simulink model "SERVER"  (R2021a)
settings: Solver=FixedStepDiscrete  StartTime=0.0  StopTime=inf  FixedStep=0.01  RelTol=1e-3  EnableMultiTasking=on
libraries: arduinolib x9, simulink x3, canmsglib x2, simulink_extras x1, dspswit3 x1
settings Model: SimulationMode=external  SILPILModeSetting=veronly  ExtModeEnableFloating=off  ExtModeTrigDuration=2  ExtModeTrigDurationFloating=2  Creator=Le Thanh Tu  LastModifiedBy=Le Thanh Tu
settings SolverCC: AlgebraicLoopSolver=TrustRegion  PositivePriorityOrder=on  AutoInsertRateTranBlk=on
settings DataIOCC: ExternalInput=[value]  SaveOutput=off  SignalLogging=off  DSMLogging=off  SaveTime=off  ReturnWorkspaceOutputs=off
settings OptimizationCC: EnhancedBackFolding=on  PassReuseOutputArgsAs=Individual arguments  ZeroExternalMemoryAtStartup=off  ZeroInternalMemoryAtStartup=off  MaxStackSize=64  OptimizeBlockOrder=speed  DifferentSizesBufferReuse=on  OptimizationCustomize=off  EfficientTunableParamExpr=on
settings DebuggingCC: ParameterTunabilityLossMsg=error  SFMachineParentedDataDiag=warning
settings HardwareCC: ProdBitPerPointer=32  ProdBitPerSizeT=32  ProdBitPerPtrDiffT=32  ProdLargestAtomicInteger=Long  ProdLargestAtomicFloat=Double  ProdWordSize=32  ProdHWDeviceType=ARM Compatible->ARM Cortex
settings SFSimCC: MATLABDynamicMemAlloc=off
settings RTWCC: SystemTargetFile=ert.tlc  HardwareBoard=Arduino Due  TemplateMakefile=ert_default_tmf  RetainRTWFile=on  Toolchain=Arduino ARM  BuildConfiguration=Faster Runs
settings CodeAppCC: ForceParamTrailComments=on  IgnoreCustomStorageClasses=off  OperatorAnnotations=on  SimulinkDataObjDesc=on  SFDataObjDesc=on  InsertBlockDesc=on
settings ERTTargetCC: SupportContinuousTime=on  SupportVariableSizeSignals=on  ExtModeStaticAllocSize=24576

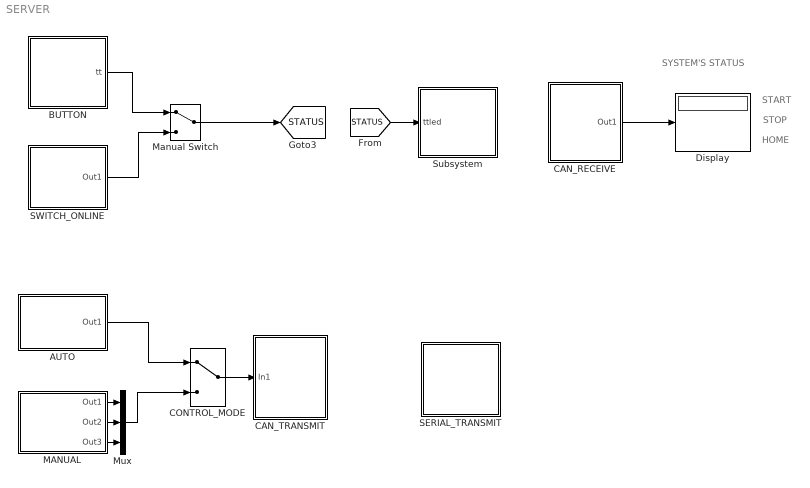
== system SERVER ==
  note: SYSTEM'S STATUS
  note: START
  note: STOP
  note: HOME
  AUTO : Subsystem
  BUTTON : Subsystem
  CAN_RECEIVE : Subsystem
  CAN_TRANSMIT : Subsystem
  CONTROL_MODE : ManualSwitch
  Display : Display
      settings: Decimation=3
  MANUAL : Subsystem
  Manual Switch : ManualSwitch
  Mux : Mux  Inputs=3
  SERIAL_TRANSMIT : Subsystem
  SWITCH_ONLINE : Subsystem
  Subsystem : Subsystem
  tag scope: STATUS=global
  wires:
  MANUAL/1(Out1) -> Mux/1
  MANUAL/2(Out2) -> Mux/2
  MANUAL/3(Out3) -> Mux/3
  Mux/1 -> CONTROL_MODE/2
  AUTO/1(Out1) -> CONTROL_MODE/1
  CAN_RECEIVE/1(Out1) -> Display/1
  SWITCH_ONLINE/1(Out1) -> Manual Switch/2
  Manual Switch/1 -> [STATUS]
  BUTTON/1(tt) -> Manual Switch/1
  CONTROL_MODE/1 -> CAN_TRANSMIT/1(In1)
  [STATUS] -> Subsystem/1(ttled)

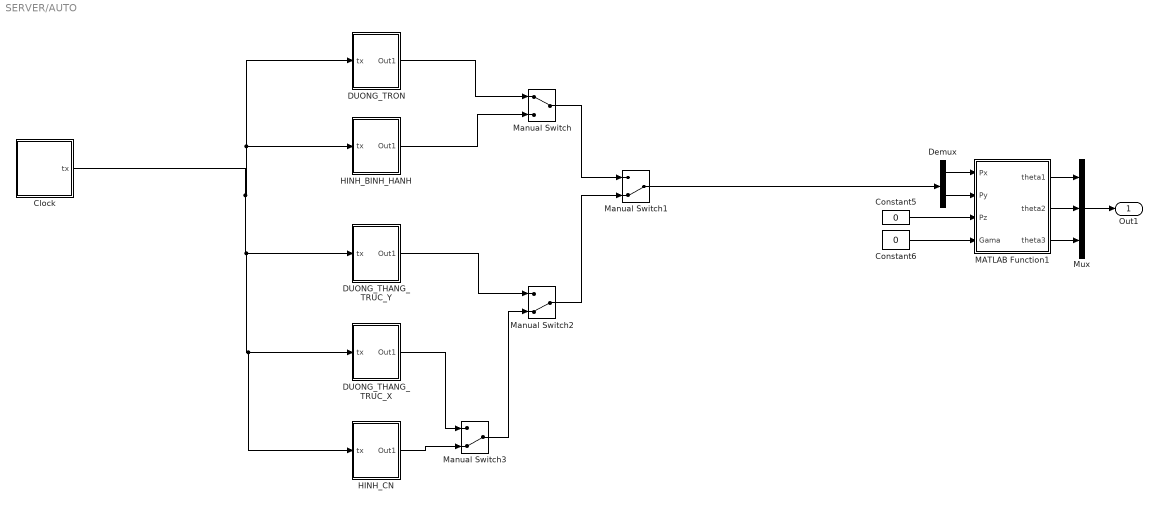
== system SERVER/AUTO ==
  Clock : Subsystem
  Constant5 : Constant  Value=0
  Constant6 : Constant  Value=0
  DUONG_THANG_TRUC_X : Subsystem
  DUONG_THANG_TRUC_Y : Subsystem
  DUONG_TRON : Subsystem
  Demux : Demux  Outputs=2
  HINH_BINH_HANH : Subsystem
  HINH_CN : Subsystem
  MATLAB Function1 : MATLAB Function  TreatAsAtomicUnit=on
  Manual Switch : ManualSwitch
  Manual Switch1 : ManualSwitch  CurrentSetting=0
  Manual Switch2 : ManualSwitch  CurrentSetting=0
  Manual Switch3 : ManualSwitch  CurrentSetting=0
  Mux : Mux  Inputs=3
  Out1 : Outport
  wires:
  HINH_BINH_HANH/1(Out1) -> Manual Switch/2
  Manual Switch2/1 -> Manual Switch1/2
  Manual Switch/1 -> Manual Switch1/1
  Demux/2 -> MATLAB Function1/2(Py)
  MATLAB Function1/3(theta3) -> Mux/3
  Demux/1 -> MATLAB Function1/1(Px)
  DUONG_TRON/1(Out1) -> Manual Switch/1
  Mux/1 -> Out1/1
  MATLAB Function1/1(theta1) -> Mux/1
  Constant5/1 -> MATLAB Function1/3(Pz)
  DUONG_THANG_TRUC_Y/1(Out1) -> Manual Switch2/1
  Constant6/1 -> MATLAB Function1/4(Gama)
  Manual Switch1/1 -> Demux/1
  MATLAB Function1/2(theta2) -> Mux/2
  Clock/1(tx) -> HINH_CN/1(tx), DUONG_THANG_TRUC_X/1(tx), DUONG_THANG_TRUC_Y/1(tx), HINH_BINH_HANH/1(tx), DUONG_TRON/1(tx)
  DUONG_THANG_TRUC_X/1(Out1) -> Manual Switch3/1
  Manual Switch3/1 -> Manual Switch2/2
  HINH_CN/1(Out1) -> Manual Switch3/2

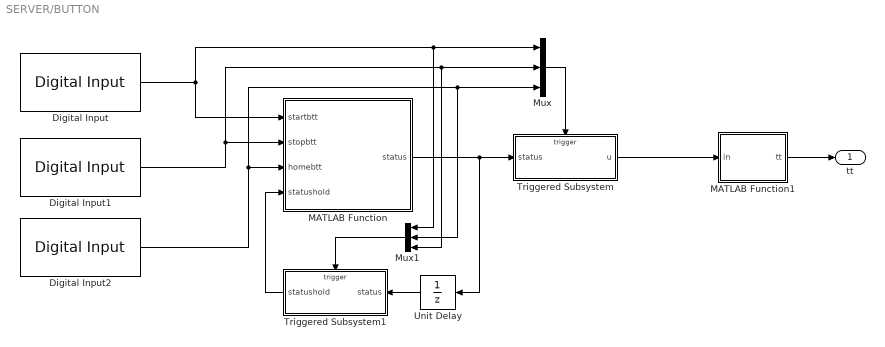
== system SERVER/BUTTON ==
  Digital Input : arduinolib/Digital Input  pinNumber=16  mode=Default  Direction=input  SampleTime=0.01  blockPlatform=arduino
  Digital Input1 : arduinolib/Digital Input  pinNumber=17  mode=Default  Direction=input  SampleTime=0.01  blockPlatform=arduino
  Digital Input2 : arduinolib/Digital Input  pinNumber=18  mode=Default  Direction=input  SampleTime=0.01  blockPlatform=arduino
  MATLAB Function : MATLAB Function  TreatAsAtomicUnit=on
  MATLAB Function1 : MATLAB Function  TreatAsAtomicUnit=on
  Mux : Mux  Inputs=3
  Mux1 : Mux  Inputs=3
  Triggered Subsystem : Subsystem  TreatAsAtomicUnit=on
  Triggered Subsystem1 : Subsystem  TreatAsAtomicUnit=on
  Unit Delay : UnitDelay  SampleTime=-1  HasFrameUpgradeWarning=on
  tt : Outport
  wires:
  Triggered Subsystem/1(u) -> MATLAB Function1/1(in)
  Digital Input2/1 -> MATLAB Function/3(homebtt), Mux1/2, Mux/3
  Unit Delay/1 -> Triggered Subsystem1/1(status)
  Mux1/1 -> Triggered Subsystem1/Trigger
  MATLAB Function/1(status) -> Unit Delay/1, Triggered Subsystem/1(status)
  MATLAB Function1/1(tt) -> tt/1
  Triggered Subsystem1/1(statushold) -> MATLAB Function/4(statushold)
  Digital Input1/1 -> MATLAB Function/2(stopbtt), Mux1/3, Mux/2
  Mux/1 -> Triggered Subsystem/Trigger
  Digital Input/1 -> MATLAB Function/1(startbtt), Mux1/1, Mux/1

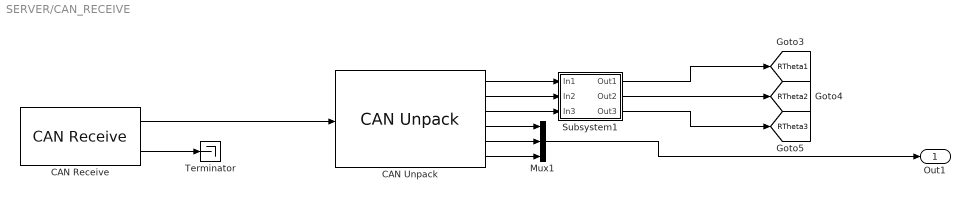
== system SERVER/CAN_RECEIVE ==
  CAN Receive : arduinolib/CAN Receive  outputDataType=CAN Msg  identifierType=Standard (11-bit identifier)  messageId=11  msgLength=6  SampleTime=0.01  outputError=off  outputRemote=off
      settings: SourceProductBaseCode=ARDUINO
  CAN Unpack : canmsglib/CAN Unpack  MsgList=(none)  MsgName=CAN Msg  MsgIDType=Standard (11-bit identifier)  MsgIdentifier=1  MsgLength=7  SignalInfo={ 'Signal1', '0', '16', 'LE', 'signed', 'Standard', '0', '1', '0', '-Inf', 'Inf'; 'Signal2', '16', '16', 'LE', 'signed', 'Standard', '0', '1', '0', '-Inf', 'Inf'; 'Signal3', '32', '16', 'LE', 'signed', 'Standard', '0', '1', '0', '-Inf', 'Inf'; 'Signal4', '48', '1', 'LE', 'unsigned', 'Standard', '0', '1', '0', '-Inf', 'Inf'; 'Signal5', '49', '1', 'LE', 'unsigned', 'Standard', '0', '1', '0', '-Inf', 'Inf'; 'Signal6', '50', '1', 'LE', 'unsigned', 'Standard', '0', '1', '0', '-Inf', 'Inf' }  IDPort=off  TimestampPort=off  ErrorPort=off  RemotePort=off  LengthPort=off  StatusPort=off  ApplyMinMax=off
      settings: SourceProductBaseCode=ME,XP,VN
  Mux1 : Mux  Inputs=3
  Subsystem1 : Subsystem
  Terminator : Terminator
  Out1 : Outport
  tag scope: RTheta1=global, RTheta2=global, RTheta3=global
  wires:
  Subsystem1/3(Out3) -> [RTheta3]
  CAN Unpack/4 -> Mux1/1
  CAN Unpack/6 -> Mux1/3
  Subsystem1/2(Out2) -> [RTheta2]
  CAN Unpack/2 -> Subsystem1/2(In2)
  CAN Receive/2 -> Terminator/1
  CAN Unpack/3 -> Subsystem1/3(In3)
  CAN Receive/1 -> CAN Unpack/1
  CAN Unpack/1 -> Subsystem1/1(In1)
  Subsystem1/1(Out1) -> [RTheta1]
  CAN Unpack/5 -> Mux1/2
  Mux1/1 -> Out1/1

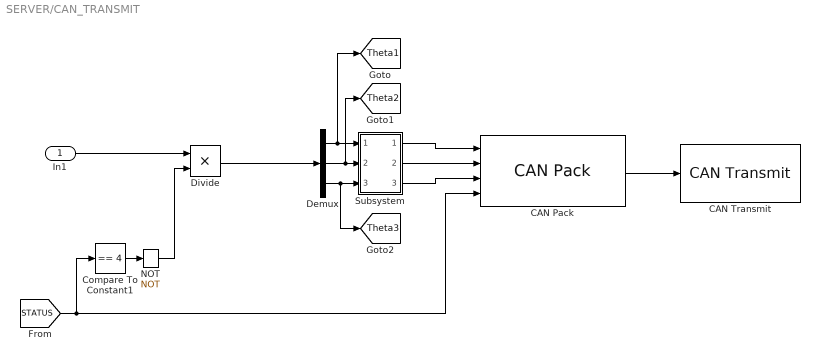
== system SERVER/CAN_TRANSMIT ==
  In1 : Inport
  CAN Pack : canmsglib/CAN Pack  MsgList=(none)  MsgName=CAN Msg  MsgIDType=Standard (11-bit identifier)  MsgIdentifier=0  MsgLength=7  Remote=off  ApplyMinMax=off  BusOutput=on  SignalInfo={ 'Signal1', '0', '16', 'LE', 'signed', 'Standard', '0', '1', '0', '-Inf', 'Inf'; 'Signal2', '16', '16', 'LE', 'signed', 'Standard', '0', '1', '0', '-Inf', 'Inf'; 'Signal3', '32', '16', 'LE', 'signed', 'Standard', '0', '1', '0', '-Inf', 'Inf'; 'Signal4', '48', '3', 'LE', 'unsigned', 'Standard', '0', '1', '0', '-Inf', 'Inf' }
      settings: SourceProductBaseCode=ME,XP,VN  DataFormat=manually specified signals
  CAN Transmit : arduinolib/CAN Transmit  inputDataType=CAN Msg  BlockingMode_=on  BlockTimeout_=0.01  outputStatus=off  identifierType=Standard (11-bit identifier)  messageId=5  msgLength=4  remoteFrame=off
      settings: SourceProductBaseCode=ARDUINO
  Compare To Constant1 : simulink/Logic and Bit Operations/Compare To Constant  relop===  const=4  OutDataTypeStr=boolean
  Demux : Demux  Outputs=3
  Divide : Product  Inputs=**
  NOT : Logic  Operator=NOT  IconShape=distinctive  AllPortsSameDT=off  OutDataTypeStr=boolean
  Subsystem : Subsystem
  tag scope: Theta1=global, Theta2=global, Theta3=global
  wires:
  Demux/2 -> [Theta2], Subsystem/2(In2)
  Subsystem/3(Out3) -> CAN Pack/3
  Demux/1 -> [Theta1], Subsystem/1(In1)
  [STATUS] -> CAN Pack/4, Compare To Constant1/1
  Demux/3 -> [Theta3], Subsystem/3(In3)
  Subsystem/2(Out2) -> CAN Pack/2
  CAN Pack/1 -> CAN Transmit/1
  Subsystem/1(Out1) -> CAN Pack/1
  Compare To Constant1/1 -> NOT/1
  NOT/1 -> Divide/2
  In1/1 -> Divide/1
  Divide/1 -> Demux/1

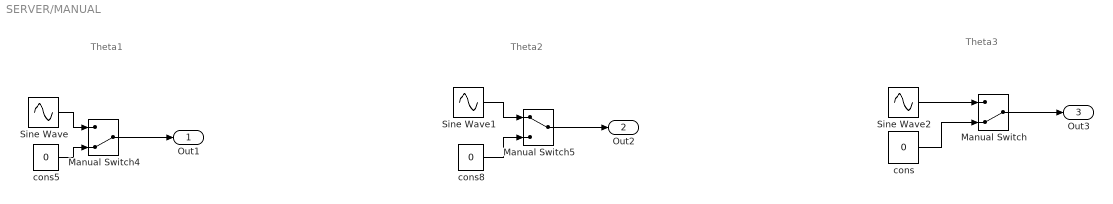
== system SERVER/MANUAL ==
  note: Theta1
  note: Theta2
  note: Theta3
  Manual Switch : ManualSwitch  CurrentSetting=0
  Manual Switch4 : ManualSwitch  CurrentSetting=0
  Manual Switch5 : ManualSwitch
  Sine Wave : Sin  Amplitude=45  Frequency=2*pi*0.05  Phase=pi/6  SampleTime=0
  Sine Wave1 : Sin  Amplitude=45  Frequency=2*pi*0.07  Phase=pi/4  SampleTime=0
  Sine Wave2 : Sin  Amplitude=90  Frequency=2*pi*0.15  Phase=pi/3  SampleTime=0
  cons : Constant  Value=0  VectorParams1D=off  OutDataTypeStr=single
  cons5 : Constant  Value=0  VectorParams1D=off  OutDataTypeStr=single
  cons8 : Constant  Value=0  VectorParams1D=off  OutDataTypeStr=single
  Out1 : Outport
  Out2 : Outport  Port=2
  Out3 : Outport  Port=3
  wires:
  Sine Wave2/1 -> Manual Switch/1
  Sine Wave1/1 -> Manual Switch5/1
  cons5/1 -> Manual Switch4/2
  cons/1 -> Manual Switch/2
  Sine Wave/1 -> Manual Switch4/1
  cons8/1 -> Manual Switch5/2
  Manual Switch5/1 -> Out2/1
  Manual Switch/1 -> Out3/1
  Manual Switch4/1 -> Out1/1

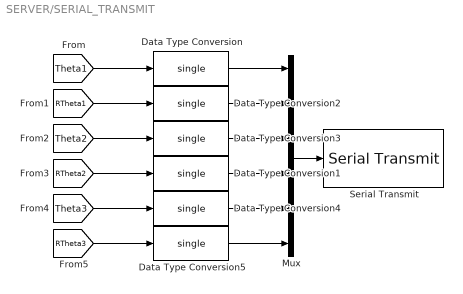
== system SERVER/SERIAL_TRANSMIT ==
  Data Type Conversion{,1..5} (6 alike) : DataTypeConversion  OutDataTypeStr=single
  Mux : Mux  Inputs=6
  Serial Transmit : arduinolib/Serial Transmit  portNumber=3  sendmode=write  label=' %f, %f, %f, %f, %f, %f;'  sendformat=Decimal  floatprecision=2  blockPlatform=arduino
  wires:
  Mux/1 -> Serial Transmit/1
  [RTheta3] -> Data Type Conversion5/1
  [Theta3] -> Data Type Conversion4/1
  [RTheta2] -> Data Type Conversion1/1
  Data Type Conversion4/1 -> Mux/5
  Data Type Conversion3/1 -> Mux/3
  Data Type Conversion/1 -> Mux/1
  [Theta1] -> Data Type Conversion/1
  Data Type Conversion1/1 -> Mux/4
  [RTheta1] -> Data Type Conversion2/1
  Data Type Conversion5/1 -> Mux/6
  [Theta2] -> Data Type Conversion3/1
  Data Type Conversion2/1 -> Mux/2

== system SERVER/SWITCH_ONLINE ==
  HOME : Subsystem
  Manual Switch6 : ManualSwitch  CurrentSetting=0
  Manual Switch7 : ManualSwitch
  START : Subsystem
  STOP : Subsystem
  Out1 : Outport
  wires:
  Manual Switch7/1 -> Manual Switch6/1
  HOME/1(Out1) -> Manual Switch6/2
  STOP/1(Out1) -> Manual Switch7/2
  START/1(Out1) -> Manual Switch7/1
  Manual Switch6/1 -> Out1/1

== system SERVER/Subsystem ==
  ttled : Inport
  Digital Output : arduinolib/Digital Output  pinNumber=19  Direction=output  blockPlatform=arduino
  Digital Output1 : arduinolib/Digital Output  pinNumber=20  Direction=output  blockPlatform=arduino
  Digital Output2 : arduinolib/Digital Output  pinNumber=21  Direction=output  blockPlatform=arduino
  MATLAB Function : MATLAB Function  TreatAsAtomicUnit=on
  wires:
  MATLAB Function/3(home) -> Digital Output2/1
  MATLAB Function/2(stop) -> Digital Output1/1
  MATLAB Function/1(start) -> Digital Output/1
  ttled/1 -> MATLAB Function/1(ttled)

== system SERVER/AUTO/Clock ==
  Clock1 : simulink_extras/Flip Flops/Clock  period=0.02
  Compare To Constant : simulink/Logic and Bit Operations/Compare To Constant  relop===  const=1  OutDataTypeStr=boolean
  Compare To Constant1 : simulink/Logic and Bit Operations/Compare To Constant  relop===  const=4  OutDataTypeStr=boolean
  Counter : dspswit3/Counter  Direction=Up  CountEvent=Either edge  CounterSize=32 bits  MaxCount=255  InitialCount=0  Output=Count  HitValue=32  ResetInput=on  SamplesPerFrame=1  Ts=1  CntDtype=double  HitDtype=Logical
  Divide : Product  Inputs=**
  Gain : Gain  Gain=0.01
  tx : Outport
  wires:
  Counter/1 -> Gain/1
  Divide/1 -> Counter/1
  Compare To Constant/1 -> Divide/1
  [STATUS] -> Compare To Constant1/1, Compare To Constant/1
  Clock1/1 -> Divide/2
  Gain/1 -> tx/1
  Compare To Constant1/1 -> Counter/2

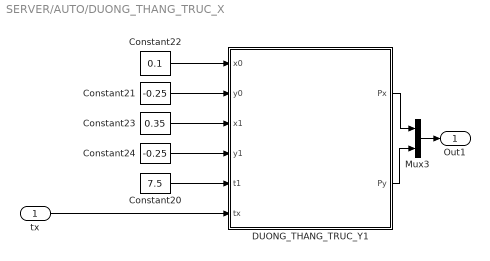
== system SERVER/AUTO/DUONG_THANG_TRUC_X ==
  tx : Inport
  Constant20 : Constant  Value=7.5
  Constant21 : Constant  Value=-0.25
  Constant22 : Constant  Value=0.1
  Constant23 : Constant  Value=0.35
  Constant24 : Constant  Value=-0.25
  DUONG_THANG_TRUC_Y1 : MATLAB Function  TreatAsAtomicUnit=on
  Mux3 : Mux  Inputs=2
  Out1 : Outport
  wires:
  Constant23/1 -> DUONG_THANG_TRUC_Y1/3(x1)
  DUONG_THANG_TRUC_Y1/2(Py) -> Mux3/2
  DUONG_THANG_TRUC_Y1/1(Px) -> Mux3/1
  Constant22/1 -> DUONG_THANG_TRUC_Y1/1(x0)
  Constant24/1 -> DUONG_THANG_TRUC_Y1/4(y1)
  tx/1 -> DUONG_THANG_TRUC_Y1/6(tx)
  Constant21/1 -> DUONG_THANG_TRUC_Y1/2(y0)
  Constant20/1 -> DUONG_THANG_TRUC_Y1/5(t1)
  Mux3/1 -> Out1/1

== system SERVER/AUTO/DUONG_THANG_TRUC_Y ==
  tx : Inport
  Constant10 : Constant  Value=7
  Constant11 : Constant  Value=0.24
  Constant7 : Constant  Value=0.33
  Constant8 : Constant  Value=0.33
  Constant9 : Constant  Value=-0.25
  DUONG_THANG_TRUC_Y : MATLAB Function  TreatAsAtomicUnit=on
  Mux2 : Mux  Inputs=2
  Out1 : Outport
  wires:
  Constant10/1 -> DUONG_THANG_TRUC_Y/5(t1)
  DUONG_THANG_TRUC_Y/2(Py) -> Mux2/2
  Constant9/1 -> DUONG_THANG_TRUC_Y/4(y1)
  Constant7/1 -> DUONG_THANG_TRUC_Y/1(x0)
  Constant11/1 -> DUONG_THANG_TRUC_Y/2(y0)
  Mux2/1 -> Out1/1
  Constant8/1 -> DUONG_THANG_TRUC_Y/3(x1)
  DUONG_THANG_TRUC_Y/1(Px) -> Mux2/1
  tx/1 -> DUONG_THANG_TRUC_Y/6(tx)

== system SERVER/AUTO/DUONG_TRON ==
  tx : Inport
  Constant : Constant  Value=0.28
  Constant1 : Constant  Value=-0.13
  Constant2 : Constant  Value=0.42
  Constant3 : Constant  Value=-0.13
  Constant4 : Constant  Value=7.5
  DUONG_TRON : MATLAB Function  TreatAsAtomicUnit=on
  Mux1 : Mux  Inputs=2
  Out1 : Outport
  wires:
  DUONG_TRON/1(Px) -> Mux1/1
  Constant/1 -> DUONG_TRON/1(x0)
  DUONG_TRON/2(Py) -> Mux1/2
  Constant1/1 -> DUONG_TRON/2(y0)
  Constant3/1 -> DUONG_TRON/4(y1)
  Constant2/1 -> DUONG_TRON/3(x1)
  Constant4/1 -> DUONG_TRON/5(t1)
  Mux1/1 -> Out1/1
  tx/1 -> DUONG_TRON/6(tx)

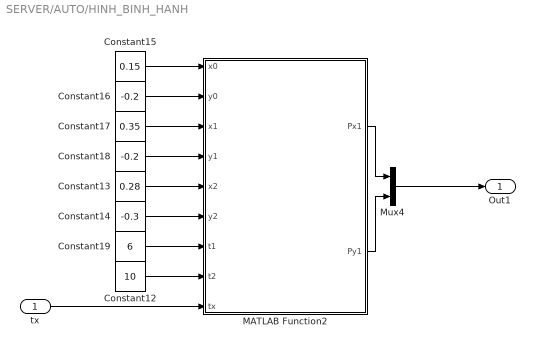
== system SERVER/AUTO/HINH_BINH_HANH ==
  tx : Inport
  Constant12 : Constant  Value=10
  Constant13 : Constant  Value=0.28
  Constant14 : Constant  Value=-0.3
  Constant15 : Constant  Value=0.15
  Constant16 : Constant  Value=-0.2
  Constant17 : Constant  Value=0.35
  Constant18 : Constant  Value=-0.2
  Constant19 : Constant  Value=6
  MATLAB Function2 : MATLAB Function  TreatAsAtomicUnit=on
  Mux4 : Mux  Inputs=2
  Out1 : Outport
  wires:
  Constant17/1 -> MATLAB Function2/3(x1)
  Constant19/1 -> MATLAB Function2/7(t1)
  Constant15/1 -> MATLAB Function2/1(x0)
  Constant14/1 -> MATLAB Function2/6(y2)
  tx/1 -> MATLAB Function2/9(tx)
  Constant13/1 -> MATLAB Function2/5(x2)
  Constant18/1 -> MATLAB Function2/4(y1)
  Constant12/1 -> MATLAB Function2/8(t2)
  Constant16/1 -> MATLAB Function2/2(y0)
  MATLAB Function2/2(Py1) -> Mux4/2
  MATLAB Function2/1(Px1) -> Mux4/1
  Mux4/1 -> Out1/1

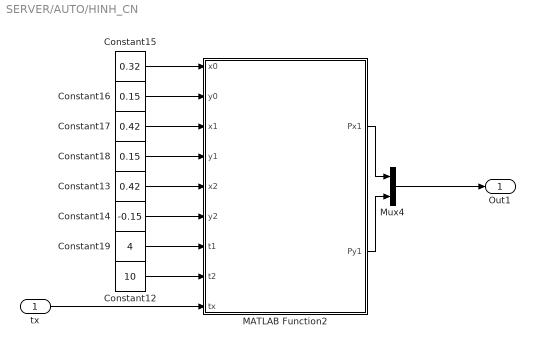
== system SERVER/AUTO/HINH_CN ==
  tx : Inport
  Constant12 : Constant  Value=10
  Constant13 : Constant  Value=0.42
  Constant14 : Constant  Value=-0.15
  Constant15 : Constant  Value=0.32
  Constant16 : Constant  Value=0.15
  Constant17 : Constant  Value=0.42
  Constant18 : Constant  Value=0.15
  Constant19 : Constant  Value=4
  MATLAB Function2 : MATLAB Function  TreatAsAtomicUnit=on
  Mux4 : Mux  Inputs=2
  Out1 : Outport
  wires:
  Mux4/1 -> Out1/1
  MATLAB Function2/1(Px1) -> Mux4/1
  MATLAB Function2/2(Py1) -> Mux4/2
  Constant16/1 -> MATLAB Function2/2(y0)
  Constant12/1 -> MATLAB Function2/8(t2)
  Constant18/1 -> MATLAB Function2/4(y1)
  Constant13/1 -> MATLAB Function2/5(x2)
  tx/1 -> MATLAB Function2/9(tx)
  Constant14/1 -> MATLAB Function2/6(y2)
  Constant15/1 -> MATLAB Function2/1(x0)
  Constant19/1 -> MATLAB Function2/7(t1)
  Constant17/1 -> MATLAB Function2/3(x1)

== system SERVER/BUTTON/Triggered Subsystem ==
  status : Inport
  Trigger : TriggerPort  VariantControl=(inherit)
  u : Outport
  wires:
  status/1 -> u/1

== system SERVER/BUTTON/Triggered Subsystem1 ==
  status : Inport
  Trigger : TriggerPort  TriggerType=either  VariantControl=(inherit)
  statushold : Outport
  wires:
  status/1 -> statushold/1

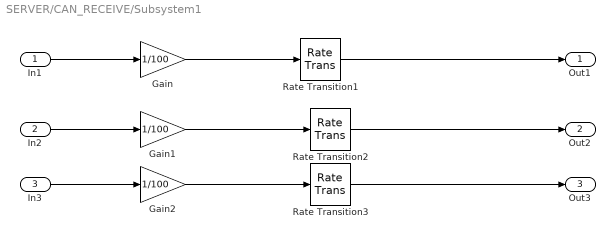
== system SERVER/CAN_RECEIVE/Subsystem1 ==
  In1 : Inport
  In2 : Inport  Port=2
  In3 : Inport  Port=3
  Gain : Gain  Gain=1/100  OutDataTypeStr=single
  Gain1 : Gain  Gain=1/100  OutDataTypeStr=single
  Gain2 : Gain  Gain=1/100
  Rate Transition1 : RateTransition  Deterministic=off
  Rate Transition2 : RateTransition  Deterministic=off
  Rate Transition3 : RateTransition  Integrity=off  Deterministic=off
  Out1 : Outport
  Out2 : Outport  Port=2
  Out3 : Outport  Port=3
  wires:
  Rate Transition2/1 -> Out2/1
  Gain2/1 -> Rate Transition3/1
  In3/1 -> Gain2/1
  Rate Transition1/1 -> Out1/1
  In2/1 -> Gain1/1
  In1/1 -> Gain/1
  Gain/1 -> Rate Transition1/1
  Gain1/1 -> Rate Transition2/1
  Rate Transition3/1 -> Out3/1

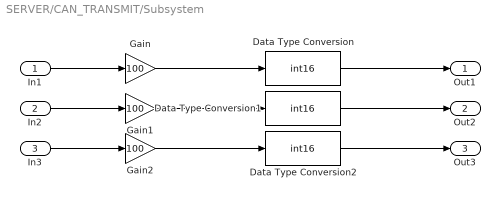
== system SERVER/CAN_TRANSMIT/Subsystem ==
  In1 : Inport
  In2 : Inport  Port=2
  In3 : Inport  Port=3
  Data Type Conversion : DataTypeConversion  OutDataTypeStr=int16
  Data Type Conversion1 : DataTypeConversion  OutDataTypeStr=int16
  Data Type Conversion2 : DataTypeConversion  OutDataTypeStr=int16
  Gain : Gain  Gain=100
  Gain1 : Gain  Gain=100
  Gain2 : Gain  Gain=100
  Out1 : Outport
  Out2 : Outport  Port=2
  Out3 : Outport  Port=3
  wires:
  Data Type Conversion2/1 -> Out3/1
  Data Type Conversion1/1 -> Out2/1
  In1/1 -> Gain/1
  Data Type Conversion/1 -> Out1/1
  In3/1 -> Gain2/1
  Gain/1 -> Data Type Conversion/1
  Gain2/1 -> Data Type Conversion2/1
  In2/1 -> Gain1/1
  Gain1/1 -> Data Type Conversion1/1

== system SERVER/SWITCH_ONLINE/HOME ==
  cons11 : Constant  Value=4  VectorParams1D=off  OutDataTypeStr=single
  Out1 : Outport
  wires:
  cons11/1 -> Out1/1

== system SERVER/SWITCH_ONLINE/START ==
  cons9 : Constant  VectorParams1D=off  OutDataTypeStr=single
  Out1 : Outport
  wires:
  cons9/1 -> Out1/1

== system SERVER/SWITCH_ONLINE/STOP ==
  cons10 : Constant  Value=2  VectorParams1D=off  OutDataTypeStr=single
  Out1 : Outport
  wires:
  cons10/1 -> Out1/1

== matlab function SERVER/Subsystem/MATLAB Function ==
  data: ttled input; start output; stop output; home output
function [start, stop, home]= fcn(ttled)
start = 0;
 stop = 0;
 home = 0;
if ttled == 4
 home = 1;
elseif ttled == 1
 start = 1;
elseif ttled == 2
 stop = 1;
else start = 0;
 stop = 0;
 home = 0;
end

== matlab function SERVER/AUTO/HINH_CN/MATLAB Function2 ==
  data: x0 input; Px1 output; y0 input; x1 input; y1 input; x2 input; y2 input; t1 input; t2 input; tx input; Py1 output
function [Px1,Py1] = fcn(x0,y0,x1,y1,x2,y2,t1,t2,tx)
v0=0;
v1=0;
t0=0;
mn= tx/t2/2;
tg = floor(mn);
t = tx - tg*t2*2;

a0x = x0;                     a0y = y0;     %canh tren
a1x = 0;                      a1y = 0;
a2x = 3*(x1-x0)/(t1^2);       a2y = 3*(y1-y0)/(t1^2);
a3x = 2*(x0-x1)/(t1^3);       a3y = 2*(y0-y1)/(t1^3);

a0x2 = x1;                    a0y2 = y1;    %canh ngang
a1x2 = 0;                     a1y2 = 0;
a2x2 = 3*(x2-x1)/((t2-t1)^2);      a2y2 = 3*(y2-y1)/((t2-t1)^2);
a3x2 = 2*(x1-x2)/((t2-t1)^3);      a3y2 = 2*(y1-y2)/((t2-t1)^3);

a0x3 = x2;                           a0y3 = y2;     %canh duoi
a1x3 = 0;                            a1y3 = 0;
a2x3 = 3*(x0-x1)/((t1)^2);       a2y3 = 3*(y0-y1)/((t1)^2);
a3x3 = 2*(x1-x0)/((t1)^3);       a3y3 = 2*(y1-y0)/((t1)^3);

%a0x4 = x2+x0-x1;                     a0y4 = y2+y0-y1;     %canh ngang cuoi
a0x4 = x2+x0-x1;                     a0y4 = y2+y0-y1; 
a1x4 = 0;                      a1y4 = 0;
a2x4 = 3*(x1-x2)/((t2-t1)^2);       a2y4 = 3*(y1-y2)/((t2-t1)^2);
a3x4 = 2*(x2-x1)/((t2-t1)^3);       a3y4 = 2*(y2-y1)/((t2-t1)^3);

if (t<=t1)
Px1 = a0x + a1x*t + a2x*t^2 + a3x*t^3;
Py1 = a0y + a1y*t + a2y*t^2 + a3y*t^3;

elseif (t1<=t)&&(t<t2)
 Px1 = a0x2 + a1x2*(t-t1) + a2x2*(t-t1)^2 + a3x2*(t-t1)^3;
Py1 = a0y2 + a1y2*(t-t1) + a2y2*(t-t1)^2 + a3y2*(t-t1)^3;
elseif (t2<= t)&&(t <= t2+t1)
   Px1 = a0x3 + a1x3*(t-t2) + a2x3*(t-t2)^2 + a3x3*(t-t2)^3;
Py1 = a0y3 + a1y3*(t-t2) + a2y3*(t-t2)^2 + a3y3*(t-t2)^3; 
%elseif (t2+t1<= t)&&(t <= t2+t1)
else
Px1 = a0x4 + a1x4*(t-t2-t1) + a2x4*(t-t2-t1)^2 + a3x4*(t-t2-t1)^3;
Py1 = a0y4 + a1y4*(t-t2-t1) + a2y4*(t-t2-t1)^2 + a3y4*(t-t2-t1)^3;
end

== matlab function SERVER/AUTO/DUONG_TRON/DUONG_TRON ==
  data: x0 input; Px output; y0 input; x1 input; y1 input; t1 input; tx input; Py output
function [Px,Py] = fcn(x0,y0,x1,y1,t1,tx)
v0=0;
v1=0;
t0=0;
mn = tx/t1/2;
tg = floor(mn);
t = tx - tg*t1*2;
Px =x0;
Py = y0;
xt = (x0+x1)/2;
yt = (y0+y1)/2;
bk = sqrt((x1-x0)^2 + (y1-y0)^2)/2;

a0x = x0;                    % a0y = y0;
a1x = 0;                     % a1y = 0;
a2x = 3*(x1-x0)/(t1^2);      % a2y = 3*(y1-y0)/(t1^2);
a3x = 2*(x0-x1)/(t1^3);      %a3y = 2*(y0-y1)/(t1^3);

a0x1 = x1;                    % a0y = y0;
a1x1 = 0;                     % a1y = 0;
a2x1 = 3*(x0-x1)/(t1^2);      % a2y = 3*(y1-y0)/(t1^2);
a3x1 = 2*(x1-x0)/(t1^3);      %a3y = 2*(y0-y1)/(t1^3);

if (t <t1)
Px = a0x + a1x*t + a2x*t^2 + a3x*t^3;
Py = (yt + sqrt(abs(bk^2 - (Px -xt)^2)));
else %if(t >=t1)&&(t <t1*2)
  Px = a0x1 + a1x1*(t-t1) + a2x1*(t-t1)^2 + a3x1*(t-t1)^3;
Py = yt - sqrt(abs(bk^2 - (Px -xt)^2));

end

== matlab function SERVER/BUTTON/MATLAB Function ==
  data: startbtt input; status output; stopbtt input; homebtt input; statushold input
function status = fcn(startbtt, stopbtt, homebtt, statushold)
status = statushold;
if (startbtt == 0)&&(statushold == 0)&&(startbtt == 0)
    status = 1;
end
if (stopbtt == 1) %%&&(homebtt == 0)   %%&&(startbtt == 1)
   if  (statushold == 1)
    status = 2;
   elseif statushold == 2
       status = 1;
   else status = statushold;
   end
end

if (homebtt == 1)&&(statushold == 1)
    status = 0;
end

== matlab function SERVER/AUTO/DUONG_THANG_TRUC_Y/DUONG_THANG_TRUC_Y ==
  data: x0 input; Px output; y0 input; x1 input; y1 input; t1 input; tx input; Py output
function [Px,Py] = fcn(x0,y0,x1,y1,t1,tx)
v0=0;
v1=0;
t0=0;
mn= tx/t1/2;
tg = floor(mn);
t = tx - tg*t1*2;
Px =x0;
Py = y0;
% xt = (x0+x1)/2;
% yt = (y0+y1)/2;
% bk = sqrt((x1-x0)^2 + (y1-y0)^2)/2;

a0x = x0;                    a0y = y0;
a1x = 0;                     a1y = 0;
a2x = 3*(x1-x0)/(t1^2);      a2y = 3*(y1-y0)/(t1^2);
a3x = 2*(x0-x1)/(t1^3);      a3y = 2*(y0-y1)/(t1^3);

a0x1 = x1;                    a0y1 = y1;
a1x1 = 0;                     a1y1 = 0;
a2x1 = 3*(x0-x1)/(t1^2);       a2y1 = 3*(y0-y1)/(t1^2);
a3x1 = 2*(x1-x0)/(t1^3);      a3y1 = 2*(y1-y0)/(t1^3);

if (t <t1)
Px = a0x + a1x*t + a2x*t^2 + a3x*t^3;
Py = a0y + a1y*t + a2y*t^2 + a3y*t^3;
%Py = (yt + sqrt(abs(bk^2 - (Px -xt)^2)));
 else %if(mod(t, t1*2) >=t1)&&(mod(t, t1*2) <t1*2)
  Px = a0x1 + a1x1*(t-t1) + a2x1*(t-t1)^2 + a3x1*(t-t1)^3;
  Py = a0y1 + a1y1*(t-t1) + a2y1*(t-t1)^2 + a3y1*(t-t1)^3;

end

== matlab function SERVER/AUTO/HINH_BINH_HANH/MATLAB Function2 ==
  data: x0 input; Px1 output; y0 input; x1 input; y1 input; x2 input; y2 input; t1 input; t2 input; tx input; Py1 output
function [Px1,Py1] = fcn(x0,y0,x1,y1,x2,y2,t1,t2,tx)
v0=0;
v1=0;
t0=0;
mn= tx/t2/2;
tg = floor(mn);
t = tx - tg*t2*2;

a0x = x0;                     a0y = y0;     %canh tren
a1x = 0;                      a1y = 0;
a2x = 3*(x1-x0)/(t1^2);       a2y = 3*(y1-y0)/(t1^2);
a3x = 2*(x0-x1)/(t1^3);       a3y = 2*(y0-y1)/(t1^3);

a0x2 = x1;                    a0y2 = y1;    %canh ngang
a1x2 = 0;                     a1y2 = 0;
a2x2 = 3*(x2-x1)/((t2-t1)^2);      a2y2 = 3*(y2-y1)/((t2-t1)^2);
a3x2 = 2*(x1-x2)/((t2-t1)^3);      a3y2 = 2*(y1-y2)/((t2-t1)^3);

a0x3 = x2;                           a0y3 = y2;     %canh duoi
a1x3 = 0;                            a1y3 = 0;
a2x3 = 3*(x0-x1)/((t1)^2);       a2y3 = 3*(y0-y1)/((t1)^2);
a3x3 = 2*(x1-x0)/((t1)^3);       a3y3 = 2*(y1-y0)/((t1)^3);

%a0x4 = x2+x0-x1;                     a0y4 = y2+y0-y1;     %canh ngang cuoi
a0x4 = x2+x0-x1;                     a0y4 = y2+y0-y1; 
a1x4 = 0;                      a1y4 = 0;
a2x4 = 3*(x1-x2)/((t2-t1)^2);       a2y4 = 3*(y1-y2)/((t2-t1)^2);
a3x4 = 2*(x2-x1)/((t2-t1)^3);       a3y4 = 2*(y2-y1)/((t2-t1)^3);

if (t<=t1)
Px1 = a0x + a1x*t + a2x*t^2 + a3x*t^3;
Py1 = a0y + a1y*t + a2y*t^2 + a3y*t^3;

elseif (t1<=t)&&(t<t2)
 Px1 = a0x2 + a1x2*(t-t1) + a2x2*(t-t1)^2 + a3x2*(t-t1)^3;
Py1 = a0y2 + a1y2*(t-t1) + a2y2*(t-t1)^2 + a3y2*(t-t1)^3;
elseif (t2<= t)&&(t <= t2+t1)
   Px1 = a0x3 + a1x3*(t-t2) + a2x3*(t-t2)^2 + a3x3*(t-t2)^3;
Py1 = a0y3 + a1y3*(t-t2) + a2y3*(t-t2)^2 + a3y3*(t-t2)^3; 
%elseif (t2+t1<= t)&&(t <= t2+t1)
else
Px1 = a0x4 + a1x4*(t-t2-t1) + a2x4*(t-t2-t1)^2 + a3x4*(t-t2-t1)^3;
Py1 = a0y4 + a1y4*(t-t2-t1) + a2y4*(t-t2-t1)^2 + a3y4*(t-t2-t1)^3;
end

== matlab function SERVER/AUTO/DUONG_THANG_TRUC_X/DUONG_THANG_TRUC_Y1 ==
  data: x0 input; Px output; y0 input; x1 input; y1 input; t1 input; tx input; Py output
function [Px,Py] = fcn(x0,y0,x1,y1,t1,tx)
v0=0;
v1=0;
t0=0;
mn= tx/t1/2;
tg = floor(mn);
t = tx - tg*t1*2;
Px =x0;
Py = y0;
% xt = (x0+x1)/2;
% yt = (y0+y1)/2;
% bk = sqrt((x1-x0)^2 + (y1-y0)^2)/2;

a0x = x0;                    a0y = y0;
a1x = 0;                     a1y = 0;
a2x = 3*(x1-x0)/(t1^2);      a2y = 3*(y1-y0)/(t1^2);
a3x = 2*(x0-x1)/(t1^3);      a3y = 2*(y0-y1)/(t1^3);

a0x1 = x1;                    a0y1 = y1;
a1x1 = 0;                     a1y1 = 0;
a2x1 = 3*(x0-x1)/(t1^2);       a2y1 = 3*(y0-y1)/(t1^2);
a3x1 = 2*(x1-x0)/(t1^3);      a3y1 = 2*(y1-y0)/(t1^3);

if (t <t1)
Px = a0x + a1x*t + a2x*t^2 + a3x*t^3;
Py = a0y + a1y*t + a2y*t^2 + a3y*t^3;
%Py = (yt + sqrt(abs(bk^2 - (Px -xt)^2)));
 else %if(mod(t, t1*2) >=t1)&&(mod(t, t1*2) <t1*2)
  Px = a0x1 + a1x1*(t-t1) + a2x1*(t-t1)^2 + a3x1*(t-t1)^3;
  Py = a0y1 + a1y1*(t-t1) + a2y1*(t-t1)^2 + a3y1*(t-t1)^3;

end

== matlab function SERVER/AUTO/MATLAB Function1 ==
  data: Px input; theta1 output; Py input; Pz input; Gama input; theta2 output; theta3 output
function [theta1, theta2, theta3] = fcn(Px, Py, Pz, Gama)
L1 = 0.17;
L2 = 0.175;
L3 = 0.125;
h= Pz;
X = Px -L3*cos(Gama);
Y = Py -L3*sin(Gama);

a = (X^2 + Y^2 - L1^2 - L2^2)/(2*L1*L2);
c = max(min(a,1),-1);
the2= -acos(c);
%the2 = 0;
theta2 = the2/pi*180;

e = atan2(Y, X);
gy = (atan2( L2*sin(the2), L1 + L2*cos(the2)));
the1 = e- gy;
theta1 = the1/pi*180;

theta3 = Gama - theta1 - theta2;

== matlab function SERVER/BUTTON/MATLAB Function1 ==
  data: in input; tt output
function tt  = fcn(in)
if in==0
  tt = 4;
elseif in == 1
   tt = 1;
elseif in == 2
   tt = 2;
else tt = 4;
end
